simulink model "test"  (R2022b)
settings: Solver=FixedStepAuto  StartTime=0.0  StopTime=50  FixedStep=0.1  RelTol=1e-3
values from neighbouring files (symbols this model uses):
  C_M = 1.1366    [init.m]
  C_T = 3.5611    [init.m]
  D_p = 0.1    [init.m]
  model_param = struct(     'I', I,      'mass', ModelParam_m,      'g', ModelParam_g,      'c_T', ModelParam_c_T,      'c_M', ModelParam_c_M,      'd', ModelParam_d,      'J_RP', ModelParam_J_RP,      'init_pos', [ModelInit_Pos_x, ModelInit_Pos_y, ModelInit_Pos_z],      'init_att', [ModelInit_Att_x, ModelInit_Att_y, ModelInit_Att_z],      'C_T', C_T,      'C_M', C_M,      'air_density', p,      'prop_diameter',  ...(+52 chars)    [init.m]
  ModelInit_Att_qw = 0    [init.m]
  ModelInit_Att_qx = 1    [init.m]
  ModelInit_Att_qy = 0    [init.m]
  ModelInit_Att_qz = 0    [init.m]
  ModelInit_Att_x = 0    [init.m]
  ModelInit_Att_y = 0    [init.m]
  ModelInit_Att_z = 0    [init.m]
  ModelInit_Pos_x = 0    [init.m]
  ModelInit_Pos_y = 0    [init.m]
  ModelInit_Pos_z = 0    [init.m]
  ModelParam_c_M = 1.779e-07*2    (= 3.558e-07)    [init.m]
  ModelParam_c_T = 1.105e-05    [init.m]
  ModelParam_d = 0.225    [init.m]
  ModelParam_g = 9.8    [init.m]
  ModelParam_I_xx = 0.0211    [init.m]
  ModelParam_I_yy = 0.0219    [init.m]
  ModelParam_I_zz = 0.0366    [init.m]
  ModelParam_J_RP = 0.0001287    [init.m]
  ModelParam_m = 1.4    [init.m]
  p = pos(idx,:)    [draw_morecool.m]    (also in init.m = 1.225)
libraries: mpclib x1
(part 1 of 3)
settings Model: Creator=12854  LastModifiedBy=12854

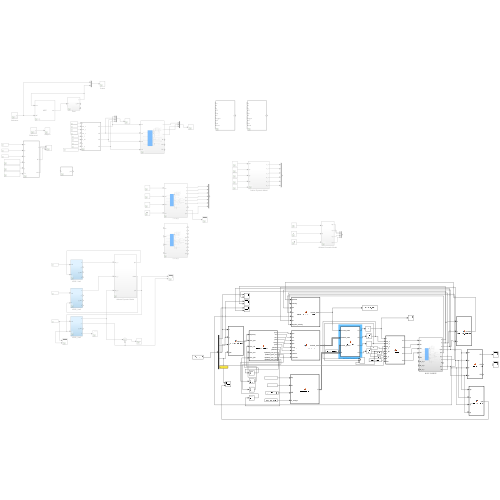
[thumbnail: Simulink's stored preview of the top-level diagram]
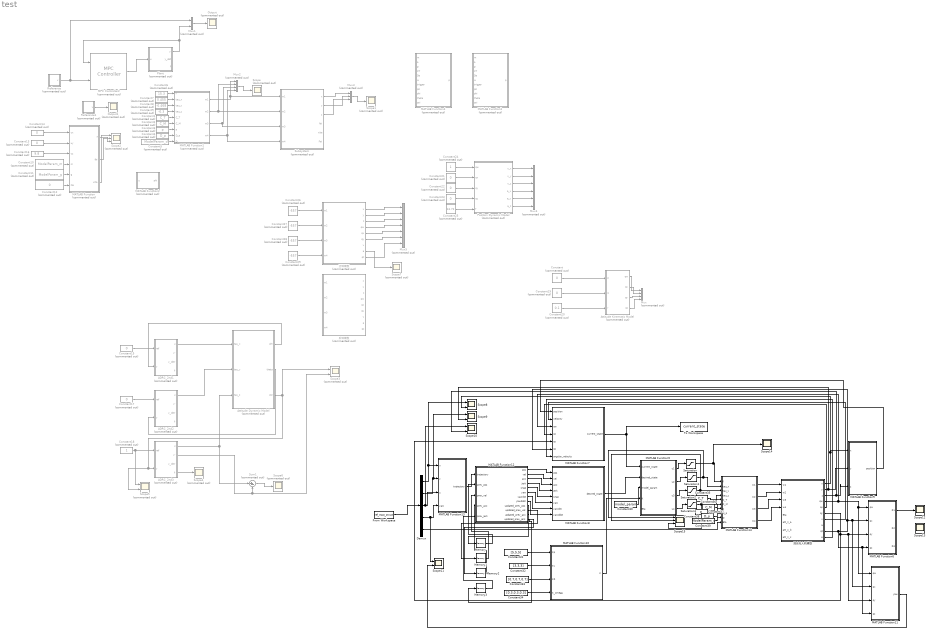
== system test ==
  ADRC_2nd1 : Subsystem  Commented=on
  ADRC_2nd2 : Subsystem  Commented=on
  ADRC_2nd3 : Subsystem  Commented=on
  Attitude Dynamic Model : Subsystem  Commented=on
  Attitude Kinematic Model : Subsystem  Commented=on
  Constant{,12..15,17,19,21..23} (10 alike) : Constant  Commented=on  Value=0
  Constant1 : Constant  Commented=on  Value=C_T
  Constant10 : Constant  Commented=on  Value=ModelParam_m
  Constant11 : Constant  Commented=on  Value=ModelParam_g
  Constant16 : Constant  Commented=on  Value=9.8
  Constant18 : Constant  Commented=on
  Constant2 : Constant  Commented=on  Value=C_M
  Constant20 : Constant  Commented=on  Value=0.1
  Constant24 : Constant  Commented=on
  Constant25 : Constant  Commented=on  Value=13.72
  Constant{26..29} (4 alike) : Constant  Commented=on  Value=-557
  Constant3 : Constant  Commented=on  Value=p
  Constant30 : Constant  Value=model_param  OutDataTypeStr=Bus: model_param_bus  SampleTime=0.1
  Constant31 : Constant  Value=[5,5,5]  SampleTime=0.1
  Constant32 : Constant  Value=[3,3,3]  SampleTime=0.1
  Constant33 : Constant  Value=[0.7,0.7,0.7]  SampleTime=0.1
  Constant34 : Constant  Value=[0.3,0.3,0.3]  SampleTime=0.1
  Constant35 : Constant  Value=C_T  SampleTime=0.1
  Constant36 : Constant  Value=C_M  SampleTime=0.1
  Constant37 : Constant  Value=p  SampleTime=0.1
  Constant38 : Constant  Value=D_p  SampleTime=0.1
  Constant39 : Constant  Value=ModelParam_d  SampleTime=0.1
  Constant4 : Constant  Commented=on  Value=D_p
  Constant5 : Constant  Commented=on  Value=ModelParam_d
  Constant6 : Constant  Commented=on  Value=15.3
  Constant7 : Constant  Commented=on  Value=0.455
  Constant8 : Constant  Commented=on  Value=-0.468
  Constant9 : Constant  Commented=on  Value=-0.3
  Demux : Demux  Outputs=5
  From Workspace : FromWorkspace  VariableName=ref_input_struct  SampleTime=0.1
  MATLAB Function : MATLAB Function  Commented=on  TreatAsAtomicUnit=on
  MATLAB Function1 : MATLAB Function  Commented=on  TreatAsAtomicUnit=on
  MATLAB Function10 : MATLAB Function  TreatAsAtomicUnit=on
  MATLAB Function11 : MATLAB Function  TreatAsAtomicUnit=on
  MATLAB Function12 : MATLAB Function  TreatAsAtomicUnit=on
  MATLAB Function13 : MATLAB Function  TreatAsAtomicUnit=on
  MATLAB Function14 : MATLAB Function  TreatAsAtomicUnit=on  SystemSampleTime=0.1
  MATLAB Function2 : MATLAB Function  Commented=on  TreatAsAtomicUnit=on
  MATLAB Function3 : MATLAB Function  Commented=on  TreatAsAtomicUnit=on
  MATLAB Function4 : MATLAB Function  Commented=on  TreatAsAtomicUnit=on
  MATLAB Function5 : MATLAB Function  TreatAsAtomicUnit=on
  MATLAB Function6 : MATLAB Function  TreatAsAtomicUnit=on
  MATLAB Function7 : MATLAB Function  TreatAsAtomicUnit=on  SystemSampleTime=0.1
  MATLAB Function8 : MATLAB Function  TreatAsAtomicUnit=on
  MATLAB Function9 : MATLAB Function  TreatAsAtomicUnit=on
  MPC Controller2 : mpclib/MPC Controller  Commented=on  SCDEnableBlockLinearizationSpecification=on  mpcobj=mpcobj  x0=[]  is_multiple=0  enable_value=0  return_u0=off  updateMPCinCallerWorkspace=on  md_inport=off  mv_inport=off  uref_inport=off  return_cost=off  return_mvseq=off  return_qpstatus=off  return_xseq=off  return_state=off  return_ovseq=off  state_inport=off  umin_inport=off  umax_inport=off  ymin_inport=off  ymax_inport=off  cc_inport=off  ywt_inport=off  uwt_inport=off  duwt_inport=off  rhoeps_inport=off  pm_inport=off  MaximumP=10  HorizonChoice=FixedHorizon  n_ts=0.1  n_p=10  n_mv=1  n_md=0  n_ud=0  n_mo=1  n_uo=0  BlockDataType=double  SampleTimeInherited=off  switch_inport=off
  Memory{,1..3} (4 alike) : Memory  InheritSampleTime=on
  Mux : Mux  Commented=on
  Mux1 : Mux  Commented=on  Inputs=2
  Mux2 : Mux  Commented=on
  Mux3 : Mux  Commented=on  Inputs=3
  Mux4 : Mux  Commented=on  Inputs=6
  Mux5 : Mux  Commented=on  Inputs=7
  Output : Scope  Commented=on
  Output1 : Scope  Commented=on
  Plant : Subsystem  Commented=on
  Position Dynamic Model : Subsystem  Commented=on
  Reference : Subsystem  Commented=on
  Reference1 : Subsystem  Commented=on
  Saturation : Saturate  UpperLimit=20  LowerLimit=0
  Saturation1 : Saturate  UpperLimit=0.3  LowerLimit=-0.3
  Saturation2 : Saturate  UpperLimit=0.3  LowerLimit=-0.3
  Saturation3 : Saturate  UpperLimit=0.3  LowerLimit=-0.3
  Scope{,1,4,6..7} (5 alike) : Scope  Commented=on
  Scope{8..11} (4 alike) : Scope  NumInputPorts=2
  Scope12 : Scope
  Scope13 : Scope
  Scope14 : Scope
  Scope15 : Scope  NumInputPorts=3
  Scope2 : Scope  Commented=on  NumInputPorts=3
  Scope3 : Scope  Commented=on  NumInputPorts=2
  Scope5 : Scope  Commented=on  NumInputPorts=2
  Subsystem : Subsystem  Commented=on
  Sum1 : Sum  Commented=on  Inputs=|+-
  To Workspace : ToWorkspace  VariableName=current_state  SaveFormat=Timeseries  SampleTime=-1
  反转模型 : Subsystem  Commented=on
  正转模型 : Subsystem  Commented=on
  混合无人机模型 : Subsystem
  wires:
  Reference/1(v) -> Mux1/1, MPC Controller2/2
  MPC Controller2/1 -> Plant/1(u)
  Plant/1(y) -> Mux1/2, MPC Controller2/1
  Mux1/1 -> Output/1
  Reference1/1(v) -> Output1/1
  Constant5/1 -> MATLAB Function1/9(D)
  Constant4/1 -> MATLAB Function1/8(D_p)
  Constant1/1 -> MATLAB Function1/5(C_T)
  Constant2/1 -> MATLAB Function1/6(C_M)
  Constant3/1 -> MATLAB Function1/7(p)
  Constant6/1 -> MATLAB Function1/1(f)
  Constant7/1 -> MATLAB Function1/2(tau_x)
  Constant8/1 -> MATLAB Function1/3(tau_y)
  Constant9/1 -> MATLAB Function1/4(tau_z)
  MATLAB Function1/1(w1) -> Subsystem/1(w1), Mux2/1
  MATLAB Function1/3(w3) -> Subsystem/3(w3), Mux2/3
  MATLAB Function1/4(w4) -> Mux2/4, Subsystem/4(w4)
  Mux2/1 -> Scope/1
  MATLAB Function1/2(w2) -> Subsystem/2(w2), Mux2/2
  Mux3/1 -> Scope1/1
  Subsystem/1(x) -> Mux3/1
  Subsystem/2(y) -> Mux3/2
  Subsystem/3(z) -> Mux3/3
  Constant10/1 -> MATLAB Function/4(m)
  Constant11/1 -> MATLAB Function/5(g)
  Constant12/1 -> MATLAB Function/6(Fai)
  Constant14/1 -> MATLAB Function/1(ux)
  Constant16/1 -> MATLAB Function/3(uz)
  MATLAB Function/1(f) -> Scope2/3
  MATLAB Function/2(fai) -> Scope2/2
  MATLAB Function/3(xita) -> Scope2/1
  Constant13/1 -> MATLAB Function/2(uy)
  ADRC_2nd1/1(u) -> Attitude Dynamic Model/1(tau_x)
  Attitude Dynamic Model/1(phi) -> ADRC_2nd1/2(y)
  Constant15/1 -> ADRC_2nd1/1(ref)
  ADRC_2nd2/1(u) -> Attitude Dynamic Model/2(tau_y)
  ADRC_2nd3/1(u) -> Sum1/1, Attitude Dynamic Model/3(tau_z)
  Attitude Dynamic Model/2(theta) -> ADRC_2nd2/2(y)
  Attitude Dynamic Model/3(psi) -> Scope5/2, ADRC_2nd3/2(y), Scope3/1
  Constant17/1 -> ADRC_2nd2/1(ref)
  Constant18/1 -> Scope5/1, ADRC_2nd3/1(ref)
  ADRC_2nd3/2(y') -> Sum1/2, Scope3/2
  ADRC_2nd3/4(f') -> Scope4/1
  Sum1/1 -> Scope6/1
  Constant/1 -> Attitude Kinematic Model/1(p)
  Constant19/1 -> Attitude Kinematic Model/2(q)
  Constant20/1 -> Attitude Kinematic Model/3(r)
  Attitude Kinematic Model/1(qw) -> Mux/1
  Attitude Kinematic Model/2(qx) -> Mux/2
  Attitude Kinematic Model/3(qy) -> Mux/3
  Attitude Kinematic Model/4(qz) -> Mux/4
  Constant21/1 -> Position Dynamic Model/2(qx)
  Constant22/1 -> Position Dynamic Model/3(qy)
  Constant23/1 -> Position Dynamic Model/4(qz)
  Constant24/1 -> Position Dynamic Model/1(qw)
  Position Dynamic Model/1(v_x) -> Mux4/1
  Position Dynamic Model/2(v_y) -> Mux4/2
  Position Dynamic Model/3(v_z) -> Mux4/3
  Position Dynamic Model/4(a_x) -> Mux4/4
  Position Dynamic Model/5(a_y) -> Mux4/5
  Position Dynamic Model/6(a_z) -> Mux4/6
  Constant25/1 -> Position Dynamic Model/5(f)
  Constant26/1 -> 正转模型/1(w1)
  Constant27/1 -> 正转模型/2(w2)
  Constant28/1 -> 正转模型/3(w3)
  Constant29/1 -> 正转模型/4(w4)
  正转模型/1(x) -> Mux5/1
  正转模型/2(y) -> Mux5/2
  正转模型/3(z) -> Mux5/3
  正转模型/4(qw) -> Mux5/4
  正转模型/5(qx) -> Mux5/5
  正转模型/6(qy) -> Mux5/6
  正转模型/9(qz) -> Mux5/7
  正转模型/8(a) -> Scope7/1
  Constant30/1 -> MATLAB Function5/3(model_param)
  Constant31/1 -> MATLAB Function10/1(Kp)
  Constant32/1 -> MATLAB Function10/2(Kv)
  Constant33/1 -> MATLAB Function10/3(KR)
  Constant34/1 -> MATLAB Function10/4(K_omega)
  MATLAB Function10/1(K) -> MATLAB Function5/4(K)
  MATLAB Function5/1(u1) -> Saturation/1
  MATLAB Function5/2(u2) -> Saturation1/1
  MATLAB Function5/3(u3) -> Saturation2/1
  MATLAB Function5/4(u4) -> Saturation3/1
  Constant35/1 -> MATLAB Function14/5(C_T)
  Constant36/1 -> MATLAB Function14/6(C_M)
  Constant37/1 -> MATLAB Function14/7(p)
  Constant38/1 -> MATLAB Function14/8(D_p)
  Constant39/1 -> MATLAB Function14/9(D)
  From Workspace/1 -> Demux/1
  Demux/5 -> MATLAB Function14/10(Eta)
  MATLAB Function14/1(w1) -> 混合无人机模型/1(w1)
  MATLAB Function14/2(w2) -> 混合无人机模型/2(w2)
  MATLAB Function14/3(w3) -> 混合无人机模型/3(w3)
  混合无人机模型/1(x) -> Scope8/2, MATLAB Function9/1(x)
  混合无人机模型/2(y) -> Scope9/2, MATLAB Function9/2(y)
  混合无人机模型/3(z) -> Scope10/2, MATLAB Function9/3(z)
  MATLAB Function9/1(position) -> MATLAB Function7/1(position)
  混合无人机模型/7(v) -> MATLAB Function7/2(velocity)
  混合无人机模型/10(w) -> MATLAB Function7/7(angular_velocity)
  混合无人机模型/4(qw) -> MATLAB Function7/3(qw), MATLAB Function11/1(qw), MATLAB Function6/1(qw)
  混合无人机模型/5(qx) -> MATLAB Function7/4(qx)
  混合无人机模型/6(qy) -> MATLAB Function11/3(qy), MATLAB Function6/3(qy), MATLAB Function7/5(qy)
  混合无人机模型/9(qz) -> MATLAB Function11/4(qz), MATLAB Function6/4(qz), MATLAB Function7/6(qz), MATLAB Function11/2(qx), MATLAB Function6/2(qx)
  MATLAB Function7/1(current_state) -> MATLAB Function5/1(current_state), To Workspace/1
  Demux/1 -> Scope8/1, MATLAB Function13/1(x)
  Demux/2 -> Scope9/1, MATLAB Function13/2(y)
  Demux/3 -> Scope10/1, MATLAB Function13/3(z)
  Demux/4 -> Scope11/1, MATLAB Function13/4(yaw)
  MATLAB Function13/1(trajectory) -> MATLAB Function12/1(trajectory)
  MATLAB Function12/1(pos) -> MATLAB Function8/1(pos)
  MATLAB Function12/2(vel) -> MATLAB Function8/2(vel)
  MATLAB Function12/3(acc) -> MATLAB Function8/3(acc)
  MATLAB Function12/4(jerk) -> MATLAB Function8/4(jerk)
  MATLAB Function12/5(snap) -> MATLAB Function8/5(snap)
  MATLAB Function12/6(yaw) -> MATLAB Function8/6(yaw)
  MATLAB Function12/7(yawdot) -> MATLAB Function8/7(yawdot)
  MATLAB Function12/8(yawddot) -> MATLAB Function8/8(yawddot)
  MATLAB Function12/9(updated_prev_pos) -> Memory/1
  Memory/1 -> MATLAB Function12/2(prev_pos)
  MATLAB Function12/10(updated_prev_vel) -> Memory1/1
  Memory1/1 -> MATLAB Function12/3(prev_vel)
  MATLAB Function12/11(updated_prev_acc) -> Memory2/1
  Memory2/1 -> MATLAB Function12/4(prev_acc)
  MATLAB Function12/12(updated_prev_jerk) -> Memory3/1
  Memory3/1 -> MATLAB Function12/5(prev_jerk)
  MATLAB Function8/1(desired_state) -> MATLAB Function5/2(desired_state)
  MATLAB Function14/4(w4) -> 混合无人机模型/4(w4)
  MATLAB Function6/1(R1) -> Scope12/1
  MATLAB Function11/1(yaw) -> Scope11/2
  Saturation/1 -> Scope14/1, MATLAB Function14/1(f)
  Saturation1/1 -> Scope15/1, MATLAB Function14/2(tau_x)
  Saturation2/1 -> Scope15/2, MATLAB Function14/3(tau_y)
  Saturation3/1 -> Scope15/3, MATLAB Function14/4(tau_z)

== system test/ADRC_2nd1 ==
  ref : Inport
  y : Inport  Port=2
  Demux : Demux  Outputs=3
  Demux1 : Demux  Outputs=2
  ESO_2nd : S-Function  FunctionName=ESO_X  Parameters=CtrlParaX  SFunctionDeploymentMode=off  EnableBusSupport=off
  Gain1 : Gain  Gain=0.0211
  Mux1 : Mux  Inputs=2
  Mux2 : Mux  Inputs=2
  NLSEF_fal_2nd : S-Function  FunctionName=NLSEF_fal_X  Parameters=CtrlParaX  SFunctionDeploymentMode=off  EnableBusSupport=off
  Sum : Sum  Inputs=|+-
  Sum1 : Sum  Inputs=|+-
  Sum2 : Sum  Inputs=|+-
  TD_2nd : S-Function  FunctionName=TD_X  Parameters=CtrlParaX  SFunctionDeploymentMode=off  EnableBusSupport=off
  u : Outport  VectorParamsAs1DForOutWhenUnconnected=off
  y' : Outport  Port=2  VectorParamsAs1DForOutWhenUnconnected=off
  y_dot' : Outport  Port=3  VectorParamsAs1DForOutWhenUnconnected=off
  f' : Outport  Port=4  VectorParamsAs1DForOutWhenUnconnected=off
  wires:
  Mux2/1 -> NLSEF_fal_2nd/1
  ESO_2nd/1 -> Demux/1
  Demux1/2 -> Sum2/1
  ref/1 -> TD_2nd/1
  Demux/1 -> y'/1, Sum1/2
  TD_2nd/1 -> Demux1/1
  y/1 -> Mux1/2
  Gain1/1 -> Sum/2
  Demux/2 -> y_dot'/1, Sum2/2
  Demux1/1 -> Sum1/1
  Demux/3 -> Gain1/1, f'/1
  Sum2/1 -> Mux2/2
  Sum/1 -> Mux1/1, u/1
  NLSEF_fal_2nd/1 -> Sum/1
  Sum1/1 -> Mux2/1
  Mux1/1 -> ESO_2nd/1

== system test/ADRC_2nd2 ==
  ref : Inport
  y : Inport  Port=2
  Demux : Demux  Outputs=3
  Demux1 : Demux  Outputs=2
  ESO_2nd : S-Function  FunctionName=ESO_Y  Parameters=CtrlParaY  SFunctionDeploymentMode=off  EnableBusSupport=off
  Gain1 : Gain  Gain=0.0219
  Mux1 : Mux  Inputs=2
  Mux2 : Mux  Inputs=2
  NLSEF_fal_2nd : S-Function  FunctionName=NLSEF_fal_Y  Parameters=CtrlParaY  SFunctionDeploymentMode=off  EnableBusSupport=off
  Sum : Sum  Inputs=|+-
  Sum1 : Sum  Inputs=|+-
  Sum2 : Sum  Inputs=|+-
  TD_2nd : S-Function  FunctionName=TD_Y  Parameters=CtrlParaY  SFunctionDeploymentMode=off  EnableBusSupport=off
  u : Outport  VectorParamsAs1DForOutWhenUnconnected=off
  y' : Outport  Port=2  VectorParamsAs1DForOutWhenUnconnected=off
  y_dot' : Outport  Port=3  VectorParamsAs1DForOutWhenUnconnected=off
  f' : Outport  Port=4  VectorParamsAs1DForOutWhenUnconnected=off
  wires:
  Mux2/1 -> NLSEF_fal_2nd/1
  ESO_2nd/1 -> Demux/1
  Demux1/2 -> Sum2/1
  ref/1 -> TD_2nd/1
  Demux/1 -> y'/1, Sum1/2
  TD_2nd/1 -> Demux1/1
  y/1 -> Mux1/2
  Gain1/1 -> Sum/2
  Demux/2 -> y_dot'/1, Sum2/2
  Demux1/1 -> Sum1/1
  Demux/3 -> Gain1/1, f'/1
  Sum2/1 -> Mux2/2
  Sum/1 -> Mux1/1, u/1
  NLSEF_fal_2nd/1 -> Sum/1
  Sum1/1 -> Mux2/1
  Mux1/1 -> ESO_2nd/1

== system test/ADRC_2nd3 ==
  ref : Inport
  y : Inport  Port=2
  Demux : Demux  Outputs=3
  Demux1 : Demux  Outputs=2
  ESO_2nd : S-Function  FunctionName=ESO_Z  Parameters=CtrlParaZ  SFunctionDeploymentMode=off  EnableBusSupport=off
  Gain1 : Gain  Gain=0.0366
  Mux1 : Mux  Inputs=2
  Mux2 : Mux  Inputs=2
  NLSEF_fal_2nd : S-Function  FunctionName=NLSEF_fal_Z  Parameters=CtrlParaZ  SFunctionDeploymentMode=off  EnableBusSupport=off
  Sum : Sum  Inputs=|+-
  Sum1 : Sum  Inputs=|+-
  Sum2 : Sum  Inputs=|+-
  TD_2nd : S-Function  FunctionName=TD_Z  Parameters=CtrlParaZ  SFunctionDeploymentMode=off  EnableBusSupport=off
  u : Outport  VectorParamsAs1DForOutWhenUnconnected=off
  y' : Outport  Port=2  VectorParamsAs1DForOutWhenUnconnected=off
  y_dot' : Outport  Port=3  VectorParamsAs1DForOutWhenUnconnected=off
  f' : Outport  Port=4  VectorParamsAs1DForOutWhenUnconnected=off
  wires:
  Mux2/1 -> NLSEF_fal_2nd/1
  ESO_2nd/1 -> Demux/1
  Demux1/2 -> Sum2/1
  ref/1 -> TD_2nd/1
  Demux/1 -> y'/1, Sum1/2
  TD_2nd/1 -> Demux1/1
  y/1 -> Mux1/2
  Gain1/1 -> Sum/2
  Demux/2 -> y_dot'/1, Sum2/2
  Demux1/1 -> Sum1/1
  Demux/3 -> Gain1/1, f'/1
  Sum2/1 -> Mux2/2
  Sum/1 -> Mux1/1, u/1
  NLSEF_fal_2nd/1 -> Sum/1
  Sum1/1 -> Mux2/1
  Mux1/1 -> ESO_2nd/1

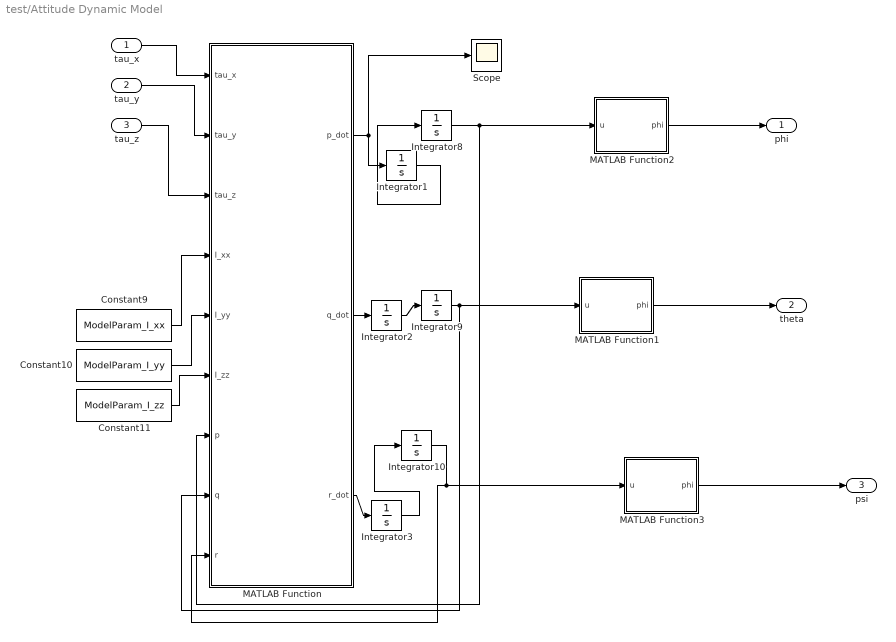
== system test/Attitude Dynamic Model ==
  tau_x : Inport
  tau_y : Inport  Port=2
  tau_z : Inport  Port=3
  Constant10 : Constant  Value=ModelParam_I_yy
  Constant11 : Constant  Value=ModelParam_I_zz
  Constant9 : Constant  Value=ModelParam_I_xx
  Integrator{1..3,8..10} (6 alike) : Integrator
  MATLAB Function : MATLAB Function  TreatAsAtomicUnit=on
  MATLAB Function1 : MATLAB Function  TreatAsAtomicUnit=on
  MATLAB Function2 : MATLAB Function  TreatAsAtomicUnit=on
  MATLAB Function3 : MATLAB Function  TreatAsAtomicUnit=on
  Scope : Scope
  phi : Outport  VectorParamsAs1DForOutWhenUnconnected=off
  theta : Outport  Port=2  VectorParamsAs1DForOutWhenUnconnected=off
  psi : Outport  Port=3  VectorParamsAs1DForOutWhenUnconnected=off
  wires:
  Constant9/1 -> MATLAB Function/4(I_xx)
  tau_z/1 -> MATLAB Function/3(tau_z)
  Integrator10/1 -> MATLAB Function3/1(u), MATLAB Function/9(r)
  Integrator9/1 -> MATLAB Function1/1(u), MATLAB Function/8(q)
  Constant10/1 -> MATLAB Function/5(I_yy)
  MATLAB Function/1(p_dot) -> Scope/1, Integrator1/1
  Integrator8/1 -> MATLAB Function2/1(u), MATLAB Function/7(p)
  tau_y/1 -> MATLAB Function/2(tau_y)
  Constant11/1 -> MATLAB Function/6(I_zz)
  tau_x/1 -> MATLAB Function/1(tau_x)
  Integrator1/1 -> Integrator8/1
  MATLAB Function/2(q_dot) -> Integrator2/1
  Integrator2/1 -> Integrator9/1
  MATLAB Function/3(r_dot) -> Integrator3/1
  Integrator3/1 -> Integrator10/1
  MATLAB Function2/1(phi) -> phi/1
  MATLAB Function1/1(phi) -> theta/1
  MATLAB Function3/1(phi) -> psi/1

== system test/Attitude Kinematic Model ==
  p : Inport
  q : Inport  Port=2
  r : Inport  Port=3
  Constant1 : Constant  Value=ModelInit_Att_qw
  Constant2 : Constant  Value=ModelInit_Att_qy
  Constant3 : Constant  Value=ModelInit_Att_qz
  Constant4 : Constant  Value=ModelInit_Att_qx
  Integrator{1,3..5} (4 alike) : Integrator  InitialConditionSource=external
  MATLAB Function2 : MATLAB Function  TreatAsAtomicUnit=on
  qw : Outport  VectorParamsAs1DForOutWhenUnconnected=off
  qx : Outport  Port=2  VectorParamsAs1DForOutWhenUnconnected=off
  qy : Outport  Port=3  VectorParamsAs1DForOutWhenUnconnected=off
  qz : Outport  Port=4  VectorParamsAs1DForOutWhenUnconnected=off
  wires:
  r/1 -> MATLAB Function2/3(r)
  MATLAB Function2/1(qw_dot) -> Integrator3/1
  q/1 -> MATLAB Function2/2(q)
  p/1 -> MATLAB Function2/1(p)
  Constant1/1 -> Integrator3/2
  Constant2/1 -> Integrator4/2
  Constant3/1 -> Integrator5/2
  Integrator3/1 -> MATLAB Function2/4(qw), qw/1
  MATLAB Function2/2(qx_dot) -> Integrator1/1
  Integrator1/1 -> MATLAB Function2/5(qx), qx/1
  Constant4/1 -> Integrator1/2
  MATLAB Function2/3(qy_dot) -> Integrator4/1
  Integrator4/1 -> MATLAB Function2/6(qy), qy/1
  MATLAB Function2/4(qz_dot) -> Integrator5/1
  Integrator5/1 -> MATLAB Function2/7(qz), qz/1

== system test/Plant ==
  u : Inport
  Clock : Clock
  Integrator : Integrator
  Integrator1 : Integrator
  MATLAB Function : MATLAB Function  TreatAsAtomicUnit=on
  To Workspace : ToWorkspace  VariableName=t  SampleTime=-1
  y : Outport  VectorParamsAs1DForOutWhenUnconnected=off
  y_dot : Outport  Port=2  VectorParamsAs1DForOutWhenUnconnected=off
  f : Outport  Port=3  VectorParamsAs1DForOutWhenUnconnected=off
  wires:
  u/1 -> MATLAB Function/2(u)
  MATLAB Function/2(x1_dot) -> Integrator/1
  MATLAB Function/1(f) -> f/1
  Integrator1/1 -> MATLAB Function/3(x2), y_dot/1
  MATLAB Function/3(x2_dot) -> Integrator1/1
  Integrator/1 -> y/1
  Clock/1 -> To Workspace/1, MATLAB Function/1(t)

== system test/Position Dynamic Model ==
  qw : Inport
  qx : Inport  Port=2
  qy : Inport  Port=3
  qz : Inport  Port=4
  f : Inport  Port=5
  Constant7 : Constant  Value=ModelParam_m
  Constant8 : Constant  Value=ModelParam_g
  Integrator1 : Integrator
  Integrator3 : Integrator
  Integrator6 : Integrator
  MATLAB Function : MATLAB Function  TreatAsAtomicUnit=on
  v_x : Outport  VectorParamsAs1DForOutWhenUnconnected=off
  v_y : Outport  Port=2  VectorParamsAs1DForOutWhenUnconnected=off
  v_z : Outport  Port=3  VectorParamsAs1DForOutWhenUnconnected=off
  a_x : Outport  Port=4  VectorParamsAs1DForOutWhenUnconnected=off
  a_y : Outport  Port=5  VectorParamsAs1DForOutWhenUnconnected=off
  a_z : Outport  Port=6  VectorParamsAs1DForOutWhenUnconnected=off
  wires:
  Constant8/1 -> MATLAB Function/2(g)
  MATLAB Function/1(v_x_dot) -> a_x/1, Integrator6/1
  MATLAB Function/2(v_y_dot) -> a_y/1, Integrator1/1
  qx/1 -> MATLAB Function/4(qx)
  Constant7/1 -> MATLAB Function/1(m)
  MATLAB Function/3(v_z_dot) -> a_z/1, Integrator3/1
  qw/1 -> MATLAB Function/3(qw)
  f/1 -> MATLAB Function/7(f)
  qy/1 -> MATLAB Function/5(qy)
  Integrator6/1 -> v_x/1
  Integrator1/1 -> v_y/1
  Integrator3/1 -> v_z/1
  qz/1 -> MATLAB Function/6(qz)

== system test/Reference ==
  Constant : Constant
  Constant1 : Constant  Value=-1
  Sine Wave : Sin  Frequency=0.75  SampleTime=0
  Switch : Switch  SaturateOnIntegerOverflow=off  InputSameDT=off
  v : Outport  VectorParamsAs1DForOutWhenUnconnected=off
  wires:
  Constant1/1 -> Switch/3
  Sine Wave/1 -> Switch/2
  Constant/1 -> Switch/1
  Switch/1 -> v/1

== system test/Reference1 ==
  Constant : Constant
  Constant1 : Constant  Value=-1
  Sine Wave : Sin  Frequency=0.75  SampleTime=0
  Switch : Switch  SaturateOnIntegerOverflow=off  InputSameDT=off
  v : Outport  VectorParamsAs1DForOutWhenUnconnected=off
  wires:
  Constant1/1 -> Switch/3
  Sine Wave/1 -> Switch/2
  Constant/1 -> Switch/1
  Switch/1 -> v/1

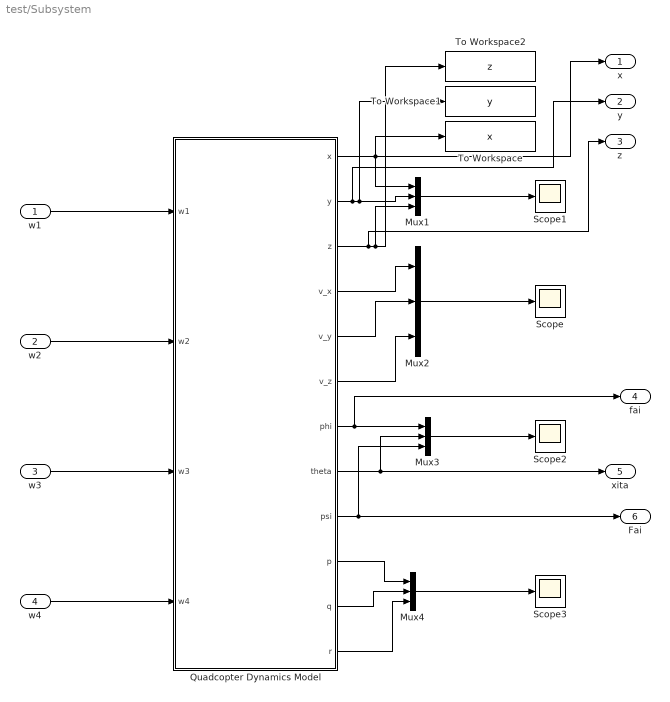
== system test/Subsystem ==
  w1 : Inport
  w2 : Inport  Port=2
  w3 : Inport  Port=3
  w4 : Inport  Port=4
  Mux{1..4} (4 alike) : Mux  Inputs=3
  Quadcopter Dynamics Model : Subsystem
  Scope{,1..3} (4 alike) : Scope
  To Workspace : ToWorkspace  VariableName=x  SaveFormat=Timeseries  SampleTime=-1
  To Workspace1 : ToWorkspace  VariableName=y  SaveFormat=Timeseries  SampleTime=-1
  To Workspace2 : ToWorkspace  VariableName=z  SaveFormat=Timeseries  SampleTime=-1
  x : Outport
  y : Outport  Port=2
  z : Outport  Port=3
  fai : Outport  Port=4
  xita : Outport  Port=5
  Fai : Outport  Port=6
  wires:
  Mux4/1 -> Scope3/1
  Mux3/1 -> Scope2/1
  Quadcopter Dynamics Model/2(y) -> y/1, To Workspace1/1, Mux1/2
  Quadcopter Dynamics Model/8(theta) -> xita/1, Mux3/2
  Quadcopter Dynamics Model/5(v_y) -> Mux2/2
  Quadcopter Dynamics Model/1(x) -> x/1, To Workspace/1, Mux1/1
  Quadcopter Dynamics Model/6(v_z) -> Mux2/3
  Mux2/1 -> Scope/1
  Quadcopter Dynamics Model/12(r) -> Mux4/3
  Mux1/1 -> Scope1/1
  Quadcopter Dynamics Model/10(p) -> Mux4/1
  Quadcopter Dynamics Model/4(v_x) -> Mux2/1
  Quadcopter Dynamics Model/7(phi) -> fai/1, Mux3/1
  Quadcopter Dynamics Model/3(z) -> z/1, To Workspace2/1, Mux1/3
  Quadcopter Dynamics Model/11(q) -> Mux4/2
  Quadcopter Dynamics Model/9(psi) -> Fai/1, Mux3/3
  w1/1 -> Quadcopter Dynamics Model/1(w1)
  w2/1 -> Quadcopter Dynamics Model/2(w2)
  w3/1 -> Quadcopter Dynamics Model/3(w3)
  w4/1 -> Quadcopter Dynamics Model/4(w4)

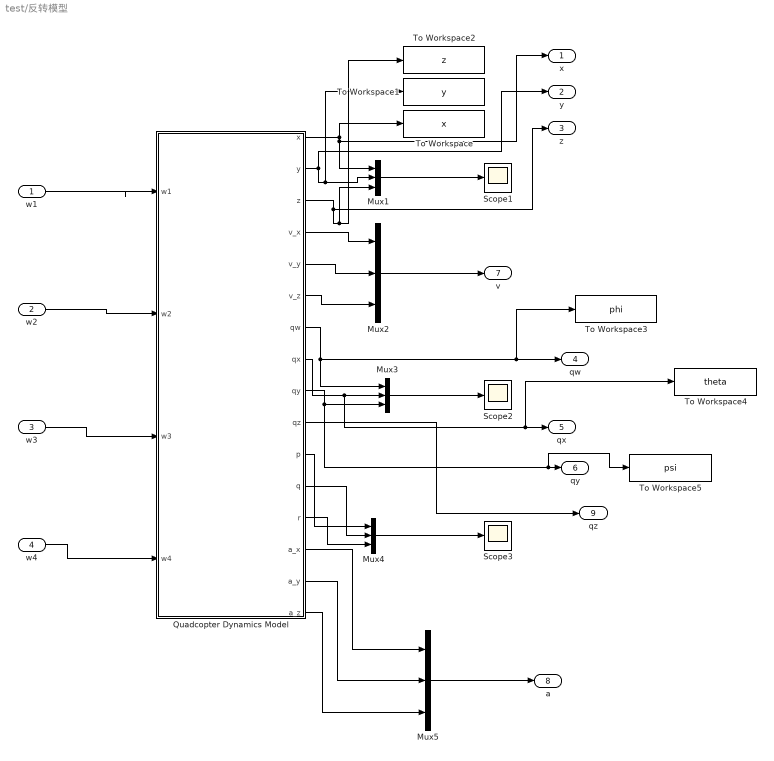
== system test/反转模型 ==
  w1 : Inport
  w2 : Inport  Port=2
  w3 : Inport  Port=3
  w4 : Inport  Port=4
  Mux{1..5} (5 alike) : Mux  Inputs=3
  Quadcopter Dynamics Model : Subsystem
  Scope1 : Scope
  Scope2 : Scope
  Scope3 : Scope
  To Workspace : ToWorkspace  VariableName=x  SaveFormat=Timeseries  SampleTime=-1
  To Workspace1 : ToWorkspace  VariableName=y  SaveFormat=Timeseries  SampleTime=-1
  To Workspace2 : ToWorkspace  VariableName=z  SaveFormat=Timeseries  SampleTime=-1
  To Workspace3 : ToWorkspace  VariableName=phi  SaveFormat=Timeseries  SampleTime=-1
  To Workspace4 : ToWorkspace  VariableName=theta  SaveFormat=Timeseries  SampleTime=-1
  To Workspace5 : ToWorkspace  VariableName=psi  SaveFormat=Timeseries  SampleTime=-1
  x : Outport
  y : Outport  Port=2
  z : Outport  Port=3
  qw : Outport  Port=4
  qx : Outport  Port=5
  qy : Outport  Port=6
  v : Outport  Port=7
  a : Outport  Port=8
  qz : Outport  Port=9
  wires:
  Mux4/1 -> Scope3/1
  Mux3/1 -> Scope2/1
  Quadcopter Dynamics Model/2(y) -> To Workspace1/1, Mux1/2, y/1
  Quadcopter Dynamics Model/8(qx) -> To Workspace4/1, qx/1, Mux3/2
  Quadcopter Dynamics Model/5(v_y) -> Mux2/2
  Quadcopter Dynamics Model/1(x) -> Mux1/1, x/1, To Workspace/1
  Quadcopter Dynamics Model/6(v_z) -> Mux2/3
  Mux2/1 -> v/1
  Quadcopter Dynamics Model/13(r) -> Mux4/3
  Mux1/1 -> Scope1/1
  Quadcopter Dynamics Model/11(p) -> Mux4/1
  Quadcopter Dynamics Model/4(v_x) -> Mux2/1
  Quadcopter Dynamics Model/7(qw) -> Mux3/1, To Workspace3/1, qw/1
  Quadcopter Dynamics Model/3(z) -> To Workspace2/1, Mux1/3, z/1
  Quadcopter Dynamics Model/12(q) -> Mux4/2
  Quadcopter Dynamics Model/9(qy) -> To Workspace5/1, qy/1, Mux3/3
  w1/1 -> Quadcopter Dynamics Model/1(w1)
  w2/1 -> Quadcopter Dynamics Model/2(w2)
  w3/1 -> Quadcopter Dynamics Model/3(w3)
  w4/1 -> Quadcopter Dynamics Model/4(w4)
  Quadcopter Dynamics Model/16(a_z) -> Mux5/3
  Quadcopter Dynamics Model/15(a_y) -> Mux5/2
  Quadcopter Dynamics Model/14(a_x) -> Mux5/1
  Mux5/1 -> a/1
  Quadcopter Dynamics Model/10(qz) -> qz/1

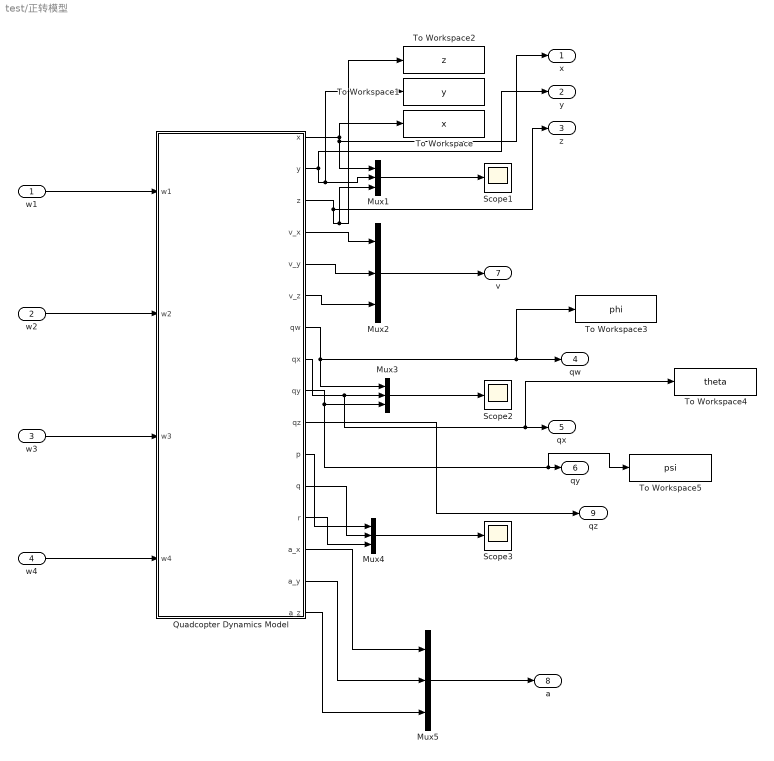
== system test/正转模型 ==
  w1 : Inport
  w2 : Inport  Port=2
  w3 : Inport  Port=3
  w4 : Inport  Port=4
  Mux{1..5} (5 alike) : Mux  Inputs=3
  Quadcopter Dynamics Model : Subsystem
  Scope1 : Scope
  Scope2 : Scope
  Scope3 : Scope
  To Workspace : ToWorkspace  VariableName=x  SaveFormat=Timeseries  SampleTime=-1
  To Workspace1 : ToWorkspace  VariableName=y  SaveFormat=Timeseries  SampleTime=-1
  To Workspace2 : ToWorkspace  VariableName=z  SaveFormat=Timeseries  SampleTime=-1
  To Workspace3 : ToWorkspace  VariableName=phi  SaveFormat=Timeseries  SampleTime=-1
  To Workspace4 : ToWorkspace  VariableName=theta  SaveFormat=Timeseries  SampleTime=-1
  To Workspace5 : ToWorkspace  VariableName=psi  SaveFormat=Timeseries  SampleTime=-1
  x : Outport
  y : Outport  Port=2
  z : Outport  Port=3
  qw : Outport  Port=4
  qx : Outport  Port=5
  qy : Outport  Port=6
  v : Outport  Port=7
  a : Outport  Port=8
  qz : Outport  Port=9
  wires:
  Mux4/1 -> Scope3/1
  Mux3/1 -> Scope2/1
  Quadcopter Dynamics Model/2(y) -> To Workspace1/1, Mux1/2, y/1
  Quadcopter Dynamics Model/8(qx) -> To Workspace4/1, qx/1, Mux3/2
  Quadcopter Dynamics Model/5(v_y) -> Mux2/2
  Quadcopter Dynamics Model/1(x) -> Mux1/1, x/1, To Workspace/1
  Quadcopter Dynamics Model/6(v_z) -> Mux2/3
  Mux2/1 -> v/1
  Quadcopter Dynamics Model/13(r) -> Mux4/3
  Mux1/1 -> Scope1/1
  Quadcopter Dynamics Model/11(p) -> Mux4/1
  Quadcopter Dynamics Model/4(v_x) -> Mux2/1
  Quadcopter Dynamics Model/7(qw) -> Mux3/1, To Workspace3/1, qw/1
  Quadcopter Dynamics Model/3(z) -> To Workspace2/1, Mux1/3, z/1
  Quadcopter Dynamics Model/12(q) -> Mux4/2
  Quadcopter Dynamics Model/9(qy) -> To Workspace5/1, qy/1, Mux3/3
  w1/1 -> Quadcopter Dynamics Model/1(w1)
  w2/1 -> Quadcopter Dynamics Model/2(w2)
  w3/1 -> Quadcopter Dynamics Model/3(w3)
  w4/1 -> Quadcopter Dynamics Model/4(w4)
  Quadcopter Dynamics Model/16(a_z) -> Mux5/3
  Quadcopter Dynamics Model/15(a_y) -> Mux5/2
  Quadcopter Dynamics Model/14(a_x) -> Mux5/1
  Mux5/1 -> a/1
  Quadcopter Dynamics Model/10(qz) -> qz/1

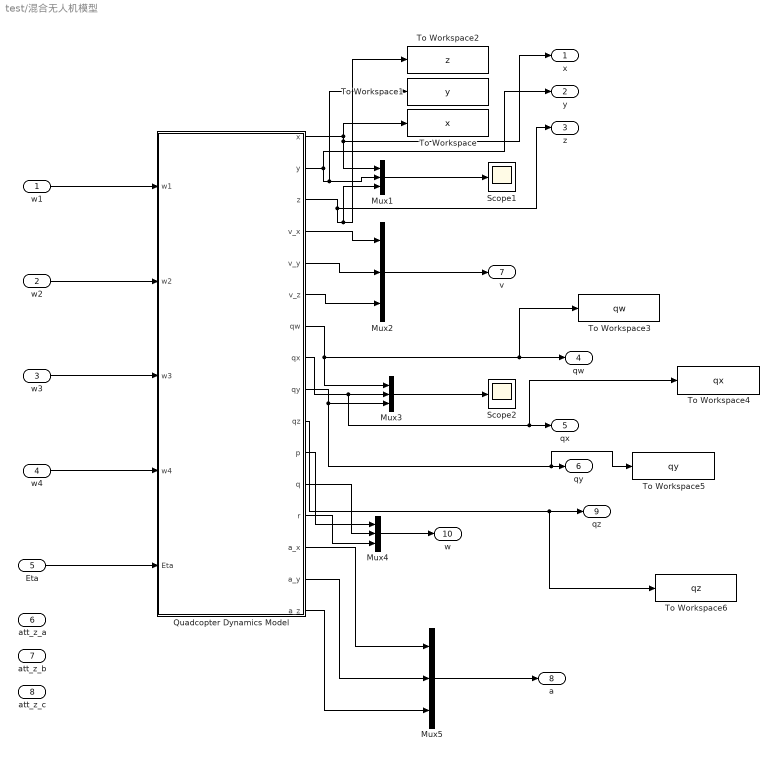
== system test/混合无人机模型 ==
  w1 : Inport
  w2 : Inport  Port=2
  w3 : Inport  Port=3
  w4 : Inport  Port=4
  Eta : Inport  Port=5
  att_z_a : Inport  Port=6
  att_z_b : Inport  Port=7
  att_z_c : Inport  Port=8
  Mux{1..5} (5 alike) : Mux  Inputs=3
  Quadcopter Dynamics Model : Subsystem
  Scope1 : Scope
  Scope2 : Scope
  To Workspace : ToWorkspace  VariableName=x  SaveFormat=Timeseries  SampleTime=-1
  To Workspace1 : ToWorkspace  VariableName=y  SaveFormat=Timeseries  SampleTime=-1
  To Workspace2 : ToWorkspace  VariableName=z  SaveFormat=Timeseries  SampleTime=-1
  To Workspace3 : ToWorkspace  VariableName=qw  SaveFormat=Timeseries  SampleTime=-1
  To Workspace4 : ToWorkspace  VariableName=qx  SaveFormat=Timeseries  SampleTime=-1
  To Workspace5 : ToWorkspace  VariableName=qy  SaveFormat=Timeseries  SampleTime=-1
  To Workspace6 : ToWorkspace  VariableName=qz  SaveFormat=Timeseries  SampleTime=-1
  x : Outport
  y : Outport  Port=2
  z : Outport  Port=3
  qw : Outport  Port=4
  qx : Outport  Port=5
  qy : Outport  Port=6
  v : Outport  Port=7
  a : Outport  Port=8
  qz : Outport  Port=9
  w : Outport  Port=10
  wires:
  Mux3/1 -> Scope2/1
  Quadcopter Dynamics Model/2(y) -> To Workspace1/1, Mux1/2, y/1
  Quadcopter Dynamics Model/8(qx) -> To Workspace4/1, qx/1, Mux3/2
  Quadcopter Dynamics Model/5(v_y) -> Mux2/2
  Quadcopter Dynamics Model/1(x) -> Mux1/1, x/1, To Workspace/1
  Quadcopter Dynamics Model/6(v_z) -> Mux2/3
  Mux2/1 -> v/1
  Quadcopter Dynamics Model/13(r) -> Mux4/3
  Mux1/1 -> Scope1/1
  Quadcopter Dynamics Model/11(p) -> Mux4/1
  Quadcopter Dynamics Model/4(v_x) -> Mux2/1
  Quadcopter Dynamics Model/7(qw) -> Mux3/1, To Workspace3/1, qw/1
  Quadcopter Dynamics Model/3(z) -> To Workspace2/1, Mux1/3, z/1
  Quadcopter Dynamics Model/12(q) -> Mux4/2
  Quadcopter Dynamics Model/9(qy) -> To Workspace5/1, qy/1, Mux3/3
  w1/1 -> Quadcopter Dynamics Model/1(w1)
  w2/1 -> Quadcopter Dynamics Model/2(w2)
  w3/1 -> Quadcopter Dynamics Model/3(w3)
  w4/1 -> Quadcopter Dynamics Model/4(w4)
  Quadcopter Dynamics Model/16(a_z) -> Mux5/3
  Quadcopter Dynamics Model/15(a_y) -> Mux5/2
  Quadcopter Dynamics Model/14(a_x) -> Mux5/1
  Mux5/1 -> a/1
  Quadcopter Dynamics Model/10(qz) -> To Workspace6/1, qz/1
  Eta/1 -> Quadcopter Dynamics Model/5(Eta)
  Mux4/1 -> w/1

== system test/Subsystem/Quadcopter Dynamics Model ==
  w1 : Inport
  w2 : Inport  Port=2
  w3 : Inport  Port=3
  w4 : Inport  Port=4
  Control Effectiveness Model : Subsystem
  Rigid-Body Dynamic Model : Subsystem
  Rigid-Body Kinematic Model : Subsystem
  x : Outport  VectorParamsAs1DForOutWhenUnconnected=off
  y : Outport  Port=2  VectorParamsAs1DForOutWhenUnconnected=off
  z : Outport  Port=3  VectorParamsAs1DForOutWhenUnconnected=off
  v_x : Outport  Port=4  VectorParamsAs1DForOutWhenUnconnected=off
  v_y : Outport  Port=5  VectorParamsAs1DForOutWhenUnconnected=off
  v_z : Outport  Port=6  VectorParamsAs1DForOutWhenUnconnected=off
  phi : Outport  Port=7  VectorParamsAs1DForOutWhenUnconnected=off
  theta : Outport  Port=8  VectorParamsAs1DForOutWhenUnconnected=off
  psi : Outport  Port=9  VectorParamsAs1DForOutWhenUnconnected=off
  p : Outport  Port=10  VectorParamsAs1DForOutWhenUnconnected=off
  q : Outport  Port=11  VectorParamsAs1DForOutWhenUnconnected=off
  r : Outport  Port=12  VectorParamsAs1DForOutWhenUnconnected=off
  wires:
  w1/1 -> Rigid-Body Dynamic Model/8(w1), Control Effectiveness Model/1(w1)
  Control Effectiveness Model/1(f) -> Rigid-Body Dynamic Model/4(f)
  w3/1 -> Rigid-Body Dynamic Model/10(w3), Control Effectiveness Model/3(w3)
  Rigid-Body Kinematic Model/5(theta) -> theta/1, Rigid-Body Dynamic Model/2(theta)
  w4/1 -> Rigid-Body Dynamic Model/11(w4), Control Effectiveness Model/4(w4)
  Rigid-Body Kinematic Model/4(phi) -> Rigid-Body Dynamic Model/1(phi), phi/1
  w2/1 -> Rigid-Body Dynamic Model/9(w2), Control Effectiveness Model/2(w2)
  Rigid-Body Dynamic Model/4(p) -> Rigid-Body Kinematic Model/4(p), p/1
  Rigid-Body Dynamic Model/3(v_z) -> Rigid-Body Kinematic Model/3(v_z), v_z/1
  Rigid-Body Dynamic Model/6(r) -> Rigid-Body Kinematic Model/6(r), r/1
  Control Effectiveness Model/2(tau_x) -> Rigid-Body Dynamic Model/5(tau_x)
  Rigid-Body Dynamic Model/2(v_y) -> Rigid-Body Kinematic Model/2(v_y), v_y/1
  Rigid-Body Kinematic Model/1(x) -> x/1
  Rigid-Body Kinematic Model/6(psi) -> psi/1, Rigid-Body Dynamic Model/3(psi)
  Rigid-Body Dynamic Model/5(q) -> Rigid-Body Kinematic Model/5(q), q/1
  Control Effectiveness Model/4(tau_z) -> Rigid-Body Dynamic Model/7(tau_z)
  Rigid-Body Kinematic Model/2(y) -> y/1
  Rigid-Body Kinematic Model/3(z) -> z/1
  Rigid-Body Dynamic Model/1(v_x) -> v_x/1, Rigid-Body Kinematic Model/1(v_x)
  Control Effectiveness Model/3(tau_y) -> Rigid-Body Dynamic Model/6(tau_y)

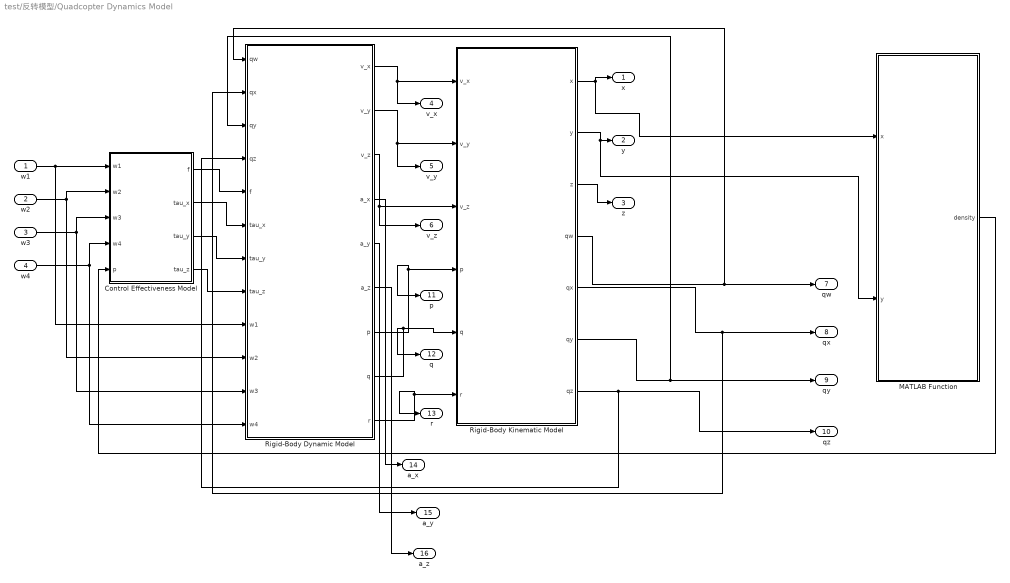
== system test/反转模型/Quadcopter Dynamics Model ==
  w1 : Inport
  w2 : Inport  Port=2
  w3 : Inport  Port=3
  w4 : Inport  Port=4
  Control Effectiveness Model : Subsystem
  MATLAB Function : MATLAB Function  TreatAsAtomicUnit=on
  Rigid-Body Dynamic Model : Subsystem
  Rigid-Body Kinematic Model : Subsystem
  x : Outport  VectorParamsAs1DForOutWhenUnconnected=off
  y : Outport  Port=2  VectorParamsAs1DForOutWhenUnconnected=off
  z : Outport  Port=3  VectorParamsAs1DForOutWhenUnconnected=off
  v_x : Outport  Port=4  VectorParamsAs1DForOutWhenUnconnected=off
  v_y : Outport  Port=5  VectorParamsAs1DForOutWhenUnconnected=off
  v_z : Outport  Port=6  VectorParamsAs1DForOutWhenUnconnected=off
  qw : Outport  Port=7  VectorParamsAs1DForOutWhenUnconnected=off
  qx : Outport  Port=8  VectorParamsAs1DForOutWhenUnconnected=off
  qy : Outport  Port=9  VectorParamsAs1DForOutWhenUnconnected=off
  qz : Outport  Port=10  VectorParamsAs1DForOutWhenUnconnected=off
  p : Outport  Port=11  VectorParamsAs1DForOutWhenUnconnected=off
  q : Outport  Port=12  VectorParamsAs1DForOutWhenUnconnected=off
  r : Outport  Port=13  VectorParamsAs1DForOutWhenUnconnected=off
  a_x : Outport  Port=14  VectorParamsAs1DForOutWhenUnconnected=off
  a_y : Outport  Port=15  VectorParamsAs1DForOutWhenUnconnected=off
  a_z : Outport  Port=16  VectorParamsAs1DForOutWhenUnconnected=off
  wires:
  w1/1 -> Rigid-Body Dynamic Model/9(w1), Control Effectiveness Model/1(w1)
  w3/1 -> Rigid-Body Dynamic Model/11(w3), Control Effectiveness Model/3(w3)
  w4/1 -> Rigid-Body Dynamic Model/12(w4), Control Effectiveness Model/4(w4)
  w2/1 -> Control Effectiveness Model/2(w2), Rigid-Body Dynamic Model/10(w2)
  Rigid-Body Dynamic Model/7(p) -> p/1, Rigid-Body Kinematic Model/4(p)
  Rigid-Body Dynamic Model/9(r) -> r/1, Rigid-Body Kinematic Model/6(r)
  Control Effectiveness Model/2(tau_x) -> Rigid-Body Dynamic Model/6(tau_x)
  Rigid-Body Kinematic Model/1(x) -> x/1, MATLAB Function/1(x)
  Rigid-Body Dynamic Model/8(q) -> q/1, Rigid-Body Kinematic Model/5(q)
  Control Effectiveness Model/4(tau_z) -> Rigid-Body Dynamic Model/8(tau_z)
  Rigid-Body Kinematic Model/2(y) -> MATLAB Function/2(y), y/1
  Rigid-Body Kinematic Model/3(z) -> z/1
  Control Effectiveness Model/3(tau_y) -> Rigid-Body Dynamic Model/7(tau_y)
  Rigid-Body Kinematic Model/4(qw) -> Rigid-Body Dynamic Model/1(qw), qw/1
  Rigid-Body Kinematic Model/5(qx) -> Rigid-Body Dynamic Model/2(qx), qx/1
  Rigid-Body Kinematic Model/6(qy) -> Rigid-Body Dynamic Model/3(qy), qy/1
  MATLAB Function/1(density) -> Control Effectiveness Model/5(p)
  Rigid-Body Dynamic Model/4(a_x) -> a_x/1
  Rigid-Body Dynamic Model/5(a_y) -> a_y/1
  Rigid-Body Dynamic Model/6(a_z) -> a_z/1
  Rigid-Body Dynamic Model/1(v_x) -> Rigid-Body Kinematic Model/1(v_x), v_x/1
  Rigid-Body Dynamic Model/2(v_y) -> Rigid-Body Kinematic Model/2(v_y), v_y/1
  Rigid-Body Dynamic Model/3(v_z) -> Rigid-Body Kinematic Model/3(v_z), v_z/1
  Control Effectiveness Model/1(f) -> Rigid-Body Dynamic Model/5(f)
  Rigid-Body Kinematic Model/7(qz) -> Rigid-Body Dynamic Model/4(qz), qz/1

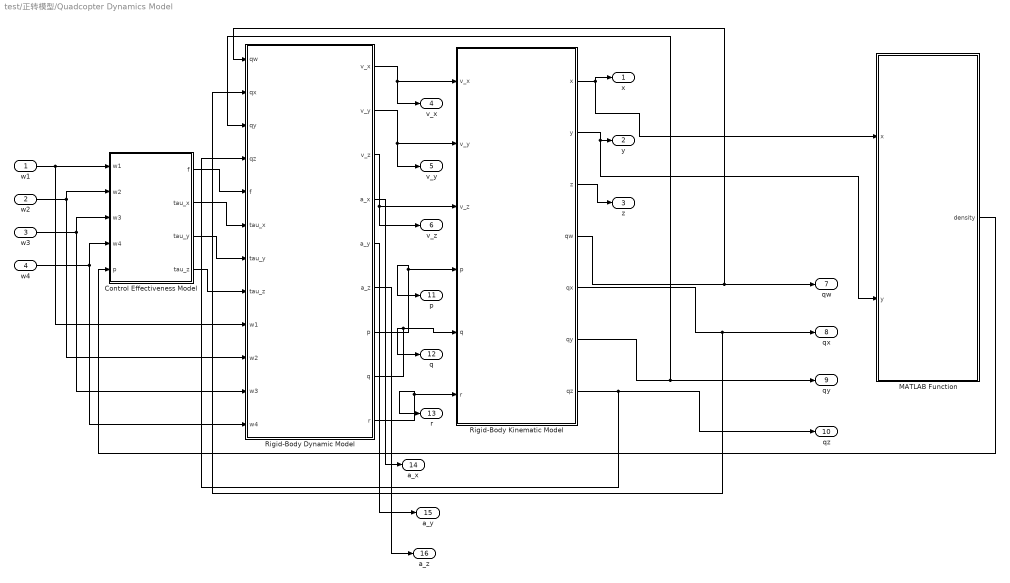
== system test/正转模型/Quadcopter Dynamics Model ==
  w1 : Inport
  w2 : Inport  Port=2
  w3 : Inport  Port=3
  w4 : Inport  Port=4
  Control Effectiveness Model : Subsystem
  MATLAB Function : MATLAB Function  TreatAsAtomicUnit=on
  Rigid-Body Dynamic Model : Subsystem
  Rigid-Body Kinematic Model : Subsystem
  x : Outport  VectorParamsAs1DForOutWhenUnconnected=off
  y : Outport  Port=2  VectorParamsAs1DForOutWhenUnconnected=off
  z : Outport  Port=3  VectorParamsAs1DForOutWhenUnconnected=off
  v_x : Outport  Port=4  VectorParamsAs1DForOutWhenUnconnected=off
  v_y : Outport  Port=5  VectorParamsAs1DForOutWhenUnconnected=off
  v_z : Outport  Port=6  VectorParamsAs1DForOutWhenUnconnected=off
  qw : Outport  Port=7  VectorParamsAs1DForOutWhenUnconnected=off
  qx : Outport  Port=8  VectorParamsAs1DForOutWhenUnconnected=off
  qy : Outport  Port=9  VectorParamsAs1DForOutWhenUnconnected=off
  qz : Outport  Port=10  VectorParamsAs1DForOutWhenUnconnected=off
  p : Outport  Port=11  VectorParamsAs1DForOutWhenUnconnected=off
  q : Outport  Port=12  VectorParamsAs1DForOutWhenUnconnected=off
  r : Outport  Port=13  VectorParamsAs1DForOutWhenUnconnected=off
  a_x : Outport  Port=14  VectorParamsAs1DForOutWhenUnconnected=off
  a_y : Outport  Port=15  VectorParamsAs1DForOutWhenUnconnected=off
  a_z : Outport  Port=16  VectorParamsAs1DForOutWhenUnconnected=off
  wires:
  w1/1 -> Rigid-Body Dynamic Model/9(w1), Control Effectiveness Model/1(w1)
  w3/1 -> Rigid-Body Dynamic Model/11(w3), Control Effectiveness Model/3(w3)
  w4/1 -> Rigid-Body Dynamic Model/12(w4), Control Effectiveness Model/4(w4)
  w2/1 -> Control Effectiveness Model/2(w2), Rigid-Body Dynamic Model/10(w2)
  Rigid-Body Dynamic Model/7(p) -> p/1, Rigid-Body Kinematic Model/4(p)
  Rigid-Body Dynamic Model/9(r) -> r/1, Rigid-Body Kinematic Model/6(r)
  Control Effectiveness Model/2(tau_x) -> Rigid-Body Dynamic Model/6(tau_x)
  Rigid-Body Kinematic Model/1(x) -> x/1, MATLAB Function/1(x)
  Rigid-Body Dynamic Model/8(q) -> q/1, Rigid-Body Kinematic Model/5(q)
  Control Effectiveness Model/4(tau_z) -> Rigid-Body Dynamic Model/8(tau_z)
  Rigid-Body Kinematic Model/2(y) -> MATLAB Function/2(y), y/1
  Rigid-Body Kinematic Model/3(z) -> z/1
  Control Effectiveness Model/3(tau_y) -> Rigid-Body Dynamic Model/7(tau_y)
  Rigid-Body Kinematic Model/4(qw) -> Rigid-Body Dynamic Model/1(qw), qw/1
  Rigid-Body Kinematic Model/5(qx) -> Rigid-Body Dynamic Model/2(qx), qx/1
  Rigid-Body Kinematic Model/6(qy) -> Rigid-Body Dynamic Model/3(qy), qy/1
  MATLAB Function/1(density) -> Control Effectiveness Model/5(p)
  Rigid-Body Dynamic Model/4(a_x) -> a_x/1
  Rigid-Body Dynamic Model/5(a_y) -> a_y/1
  Rigid-Body Dynamic Model/6(a_z) -> a_z/1
  Rigid-Body Dynamic Model/1(v_x) -> Rigid-Body Kinematic Model/1(v_x), v_x/1
  Rigid-Body Dynamic Model/2(v_y) -> Rigid-Body Kinematic Model/2(v_y), v_y/1
  Rigid-Body Dynamic Model/3(v_z) -> Rigid-Body Kinematic Model/3(v_z), v_z/1
  Control Effectiveness Model/1(f) -> Rigid-Body Dynamic Model/5(f)
  Rigid-Body Kinematic Model/7(qz) -> Rigid-Body Dynamic Model/4(qz), qz/1

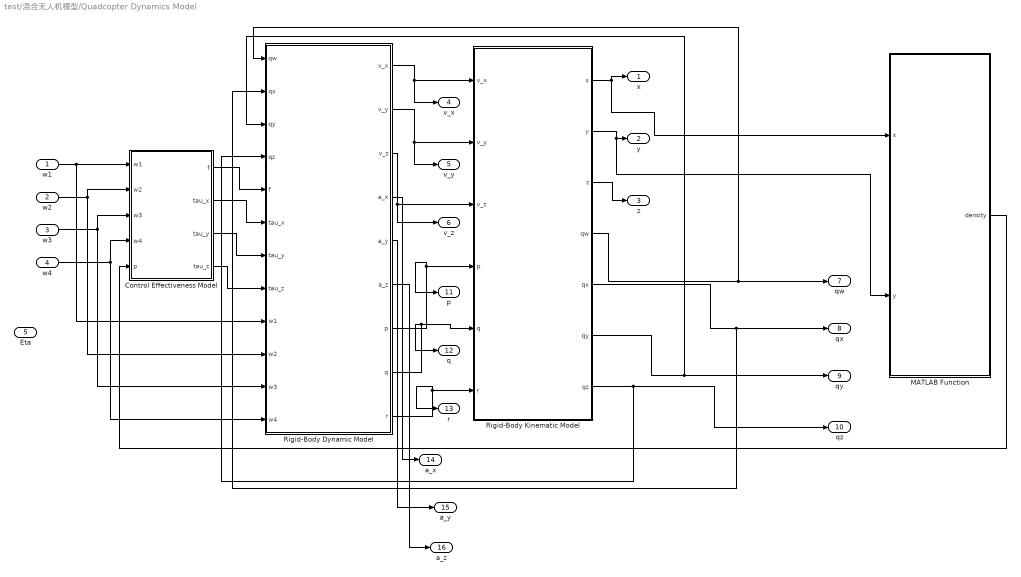
== system test/混合无人机模型/Quadcopter Dynamics Model ==
  w1 : Inport
  w2 : Inport  Port=2
  w3 : Inport  Port=3
  w4 : Inport  Port=4
  Eta : Inport  Port=5
  Control Effectiveness Model : Subsystem
  MATLAB Function : MATLAB Function  TreatAsAtomicUnit=on
  Rigid-Body Dynamic Model : Subsystem
  Rigid-Body Kinematic Model : Subsystem
  x : Outport  VectorParamsAs1DForOutWhenUnconnected=off
  y : Outport  Port=2  VectorParamsAs1DForOutWhenUnconnected=off
  z : Outport  Port=3  VectorParamsAs1DForOutWhenUnconnected=off
  v_x : Outport  Port=4  VectorParamsAs1DForOutWhenUnconnected=off
  v_y : Outport  Port=5  VectorParamsAs1DForOutWhenUnconnected=off
  v_z : Outport  Port=6  VectorParamsAs1DForOutWhenUnconnected=off
  qw : Outport  Port=7  VectorParamsAs1DForOutWhenUnconnected=off
  qx : Outport  Port=8  VectorParamsAs1DForOutWhenUnconnected=off
  qy : Outport  Port=9  VectorParamsAs1DForOutWhenUnconnected=off
  qz : Outport  Port=10  VectorParamsAs1DForOutWhenUnconnected=off
  p : Outport  Port=11  VectorParamsAs1DForOutWhenUnconnected=off
  q : Outport  Port=12  VectorParamsAs1DForOutWhenUnconnected=off
  r : Outport  Port=13  VectorParamsAs1DForOutWhenUnconnected=off
  a_x : Outport  Port=14  VectorParamsAs1DForOutWhenUnconnected=off
  a_y : Outport  Port=15  VectorParamsAs1DForOutWhenUnconnected=off
  a_z : Outport  Port=16  VectorParamsAs1DForOutWhenUnconnected=off
  wires:
  w1/1 -> Rigid-Body Dynamic Model/9(w1), Control Effectiveness Model/1(w1)
  w3/1 -> Rigid-Body Dynamic Model/11(w3), Control Effectiveness Model/3(w3)
  w4/1 -> Rigid-Body Dynamic Model/12(w4), Control Effectiveness Model/4(w4)
  w2/1 -> Control Effectiveness Model/2(w2), Rigid-Body Dynamic Model/10(w2)
  Rigid-Body Dynamic Model/7(p) -> p/1, Rigid-Body Kinematic Model/4(p)
  Rigid-Body Dynamic Model/9(r) -> r/1, Rigid-Body Kinematic Model/6(r)
  Control Effectiveness Model/2(tau_x) -> Rigid-Body Dynamic Model/6(tau_x)
  Rigid-Body Kinematic Model/1(x) -> x/1, MATLAB Function/1(x)
  Rigid-Body Dynamic Model/8(q) -> q/1, Rigid-Body Kinematic Model/5(q)
  Control Effectiveness Model/4(tau_z) -> Rigid-Body Dynamic Model/8(tau_z)
  Rigid-Body Kinematic Model/2(y) -> MATLAB Function/2(y), y/1
  Rigid-Body Kinematic Model/3(z) -> z/1
  Control Effectiveness Model/3(tau_y) -> Rigid-Body Dynamic Model/7(tau_y)
  Rigid-Body Kinematic Model/4(qw) -> Rigid-Body Dynamic Model/1(qw), qw/1
  Rigid-Body Kinematic Model/5(qx) -> Rigid-Body Dynamic Model/2(qx), qx/1
  Rigid-Body Kinematic Model/6(qy) -> Rigid-Body Dynamic Model/3(qy), qy/1
  MATLAB Function/1(density) -> Control Effectiveness Model/5(p)
  Rigid-Body Dynamic Model/4(a_x) -> a_x/1
  Rigid-Body Dynamic Model/5(a_y) -> a_y/1
  Rigid-Body Dynamic Model/6(a_z) -> a_z/1
  Rigid-Body Dynamic Model/1(v_x) -> Rigid-Body Kinematic Model/1(v_x), v_x/1
  Rigid-Body Dynamic Model/2(v_y) -> Rigid-Body Kinematic Model/2(v_y), v_y/1
  Rigid-Body Dynamic Model/3(v_z) -> Rigid-Body Kinematic Model/3(v_z), v_z/1
  Control Effectiveness Model/1(f) -> Rigid-Body Dynamic Model/5(f)
  Rigid-Body Kinematic Model/7(qz) -> Rigid-Body Dynamic Model/4(qz), qz/1

== system test/Subsystem/Quadcopter Dynamics Model/Control Effectiveness Model ==
  w1 : Inport
  w2 : Inport  Port=2
  w3 : Inport  Port=3
  w4 : Inport  Port=4
  Constant : Constant  Value=ModelParam_c_T
  Constant1 : Constant  Value=ModelParam_c_M
  Constant2 : Constant  Value=ModelParam_d
  MATLAB Function : MATLAB Function  TreatAsAtomicUnit=on
  f : Outport  VectorParamsAs1DForOutWhenUnconnected=off
  tau_x : Outport  Port=2  VectorParamsAs1DForOutWhenUnconnected=off
  tau_y : Outport  Port=3  VectorParamsAs1DForOutWhenUnconnected=off
  tau_z : Outport  Port=4  VectorParamsAs1DForOutWhenUnconnected=off
  wires:
  Constant1/1 -> MATLAB Function/6(c_M)
  Constant/1 -> MATLAB Function/5(c_T)
  MATLAB Function/3(tau_y) -> tau_y/1
  MATLAB Function/1(f) -> f/1
  Constant2/1 -> MATLAB Function/7(d)
  MATLAB Function/4(tau_z) -> tau_z/1
  w3/1 -> MATLAB Function/3(w3)
  w1/1 -> MATLAB Function/1(w1)
  w4/1 -> MATLAB Function/4(w4)
  MATLAB Function/2(tau_x) -> tau_x/1
  w2/1 -> MATLAB Function/2(w2)

== system test/Subsystem/Quadcopter Dynamics Model/Rigid-Body Dynamic Model ==
  phi : Inport
  theta : Inport  Port=2
  psi : Inport  Port=3
  f : Inport  Port=4
  tau_x : Inport  Port=5
  tau_y : Inport  Port=6
  tau_z : Inport  Port=7
  w1 : Inport  Port=8
  w2 : Inport  Port=9
  w3 : Inport  Port=10
  w4 : Inport  Port=11
  Attitude Dynamic Model : Subsystem
  Position Dynamic Model : Subsystem
  v_x : Outport  VectorParamsAs1DForOutWhenUnconnected=off
  v_y : Outport  Port=2  VectorParamsAs1DForOutWhenUnconnected=off
  v_z : Outport  Port=3  VectorParamsAs1DForOutWhenUnconnected=off
  p : Outport  Port=4  VectorParamsAs1DForOutWhenUnconnected=off
  q : Outport  Port=5  VectorParamsAs1DForOutWhenUnconnected=off
  r : Outport  Port=6  VectorParamsAs1DForOutWhenUnconnected=off
  wires:
  w3/1 -> Attitude Dynamic Model/6(w3)
  w1/1 -> Attitude Dynamic Model/4(w1)
  theta/1 -> Position Dynamic Model/2(theta)
  f/1 -> Position Dynamic Model/4(f)
  tau_x/1 -> Attitude Dynamic Model/1(tau_x)
  w2/1 -> Attitude Dynamic Model/5(w2)
  Attitude Dynamic Model/1(p) -> p/1
  w4/1 -> Attitude Dynamic Model/7(w4)
  Attitude Dynamic Model/2(q) -> q/1
  tau_y/1 -> Attitude Dynamic Model/2(tau_y)
  tau_z/1 -> Attitude Dynamic Model/3(tau_z)
  Position Dynamic Model/3(v_z) -> v_z/1
  Attitude Dynamic Model/3(r) -> r/1
  phi/1 -> Position Dynamic Model/1(phi)
  psi/1 -> Position Dynamic Model/3(psi)
  Position Dynamic Model/1(v_x) -> v_x/1
  Position Dynamic Model/2(v_y) -> v_y/1

== system test/Subsystem/Quadcopter Dynamics Model/Rigid-Body Kinematic Model ==
  v_x : Inport
  v_y : Inport  Port=2
  v_z : Inport  Port=3
  p : Inport  Port=4
  q : Inport  Port=5
  r : Inport  Port=6
  Attitude Kinematic Model : Subsystem
  Position Kinematic Model : Subsystem
  x : Outport  VectorParamsAs1DForOutWhenUnconnected=off
  y : Outport  Port=2  VectorParamsAs1DForOutWhenUnconnected=off
  z : Outport  Port=3  VectorParamsAs1DForOutWhenUnconnected=off
  phi : Outport  Port=4  VectorParamsAs1DForOutWhenUnconnected=off
  theta : Outport  Port=5  VectorParamsAs1DForOutWhenUnconnected=off
  psi : Outport  Port=6  VectorParamsAs1DForOutWhenUnconnected=off
  wires:
  v_x/1 -> Position Kinematic Model/1(v_x)
  v_y/1 -> Position Kinematic Model/2(v_y)
  r/1 -> Attitude Kinematic Model/3(r)
  p/1 -> Attitude Kinematic Model/1(p)
  v_z/1 -> Position Kinematic Model/3(v_z)
  Position Kinematic Model/1(x) -> x/1
  Position Kinematic Model/2(y) -> y/1
  q/1 -> Attitude Kinematic Model/2(q)
  Position Kinematic Model/3(z) -> z/1
  Attitude Kinematic Model/2(theta) -> theta/1
  Attitude Kinematic Model/1(phi) -> phi/1
  Attitude Kinematic Model/3(psi) -> psi/1

== system test/反转模型/Quadcopter Dynamics Model/Control Effectiveness Model ==
  w1 : Inport
  w2 : Inport  Port=2
  w3 : Inport  Port=3
  w4 : Inport  Port=4
  p : Inport  Port=5
  Constant : Constant  Value=ModelParam_c_T
  Constant1 : Constant  Value=ModelParam_c_M
  Constant2 : Constant  Value=ModelParam_d
  MATLAB Function : MATLAB Function  TreatAsAtomicUnit=on
  f : Outport  VectorParamsAs1DForOutWhenUnconnected=off
  tau_x : Outport  Port=2  VectorParamsAs1DForOutWhenUnconnected=off
  tau_y : Outport  Port=3  VectorParamsAs1DForOutWhenUnconnected=off
  tau_z : Outport  Port=4  VectorParamsAs1DForOutWhenUnconnected=off
  wires:
  Constant1/1 -> MATLAB Function/6(c_M)
  Constant/1 -> MATLAB Function/5(c_T)
  MATLAB Function/3(tau_y) -> tau_y/1
  MATLAB Function/1(f) -> f/1
  Constant2/1 -> MATLAB Function/7(d)
  MATLAB Function/4(tau_z) -> tau_z/1
  w3/1 -> MATLAB Function/3(w3)
  w1/1 -> MATLAB Function/1(w1)
  w4/1 -> MATLAB Function/4(w4)
  MATLAB Function/2(tau_x) -> tau_x/1
  w2/1 -> MATLAB Function/2(w2)
  p/1 -> MATLAB Function/8(p)

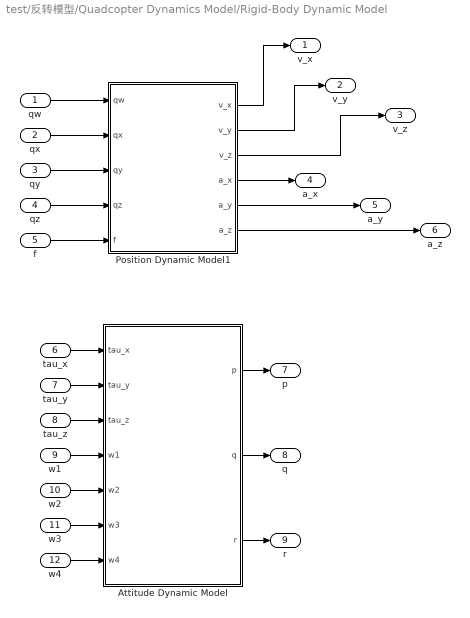
== system test/反转模型/Quadcopter Dynamics Model/Rigid-Body Dynamic Model ==
  qw : Inport
  qx : Inport  Port=2
  qy : Inport  Port=3
  qz : Inport  Port=4
  f : Inport  Port=5
  tau_x : Inport  Port=6
  tau_y : Inport  Port=7
  tau_z : Inport  Port=8
  w1 : Inport  Port=9
  w2 : Inport  Port=10
  w3 : Inport  Port=11
  w4 : Inport  Port=12
  Attitude Dynamic Model : Subsystem
  Position Dynamic Model1 : Subsystem
  v_x : Outport  VectorParamsAs1DForOutWhenUnconnected=off
  v_y : Outport  Port=2  VectorParamsAs1DForOutWhenUnconnected=off
  v_z : Outport  Port=3  VectorParamsAs1DForOutWhenUnconnected=off
  a_x : Outport  Port=4  VectorParamsAs1DForOutWhenUnconnected=off
  a_y : Outport  Port=5  VectorParamsAs1DForOutWhenUnconnected=off
  a_z : Outport  Port=6  VectorParamsAs1DForOutWhenUnconnected=off
  p : Outport  Port=7  VectorParamsAs1DForOutWhenUnconnected=off
  q : Outport  Port=8  VectorParamsAs1DForOutWhenUnconnected=off
  r : Outport  Port=9  VectorParamsAs1DForOutWhenUnconnected=off
  wires:
  w3/1 -> Attitude Dynamic Model/6(w3)
  w1/1 -> Attitude Dynamic Model/4(w1)
  tau_x/1 -> Attitude Dynamic Model/1(tau_x)
  w2/1 -> Attitude Dynamic Model/5(w2)
  Attitude Dynamic Model/1(p) -> p/1
  w4/1 -> Attitude Dynamic Model/7(w4)
  Attitude Dynamic Model/2(q) -> q/1
  tau_y/1 -> Attitude Dynamic Model/2(tau_y)
  tau_z/1 -> Attitude Dynamic Model/3(tau_z)
  Attitude Dynamic Model/3(r) -> r/1
  qw/1 -> Position Dynamic Model1/1(qw)
  qx/1 -> Position Dynamic Model1/2(qx)
  qy/1 -> Position Dynamic Model1/3(qy)
  qz/1 -> Position Dynamic Model1/4(qz)
  f/1 -> Position Dynamic Model1/5(f)
  Position Dynamic Model1/1(v_x) -> v_x/1
  Position Dynamic Model1/2(v_y) -> v_y/1
  Position Dynamic Model1/3(v_z) -> v_z/1
  Position Dynamic Model1/4(a_x) -> a_x/1
  Position Dynamic Model1/5(a_y) -> a_y/1
  Position Dynamic Model1/6(a_z) -> a_z/1

== system test/反转模型/Quadcopter Dynamics Model/Rigid-Body Kinematic Model ==
  v_x : Inport
  v_y : Inport  Port=2
  v_z : Inport  Port=3
  p : Inport  Port=4
  q : Inport  Port=5
  r : Inport  Port=6
  Attitude Kinematic Model1 : Subsystem
  Position Kinematic Model : Subsystem
  x : Outport  VectorParamsAs1DForOutWhenUnconnected=off
  y : Outport  Port=2  VectorParamsAs1DForOutWhenUnconnected=off
  z : Outport  Port=3  VectorParamsAs1DForOutWhenUnconnected=off
  qw : Outport  Port=4  VectorParamsAs1DForOutWhenUnconnected=off
  qx : Outport  Port=5  VectorParamsAs1DForOutWhenUnconnected=off
  qy : Outport  Port=6  VectorParamsAs1DForOutWhenUnconnected=off
  qz : Outport  Port=7  VectorParamsAs1DForOutWhenUnconnected=off
  wires:
  v_x/1 -> Position Kinematic Model/1(v_x)
  v_y/1 -> Position Kinematic Model/2(v_y)
  r/1 -> Attitude Kinematic Model1/3(r)
  p/1 -> Attitude Kinematic Model1/1(p)
  v_z/1 -> Position Kinematic Model/3(v_z)
  Position Kinematic Model/1(x) -> x/1
  Position Kinematic Model/2(y) -> y/1
  q/1 -> Attitude Kinematic Model1/2(q)
  Position Kinematic Model/3(z) -> z/1
  Attitude Kinematic Model1/2(qx) -> qx/1
  Attitude Kinematic Model1/1(qw) -> qw/1
  Attitude Kinematic Model1/3(qy) -> qy/1
  Attitude Kinematic Model1/4(qz) -> qz/1
